simulink subsystem "flag_LiDAR_online"  (R2024a)
settings: Solver=VariableStepAuto  StartTime=0.0  StopTime=10.0  RelTol=1e-3
settings Model: Creator=gurt1  LastModifiedBy=gurt1

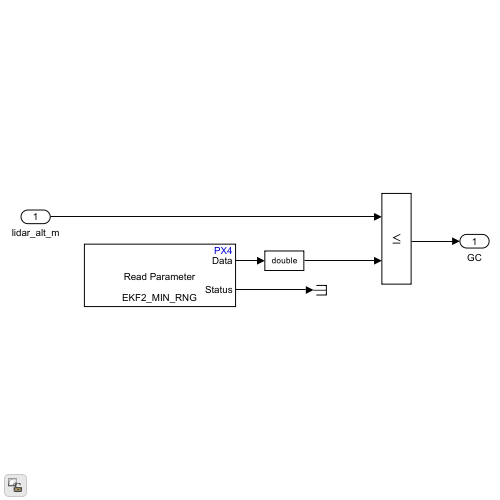
[thumbnail: Simulink's stored preview of the top-level diagram]
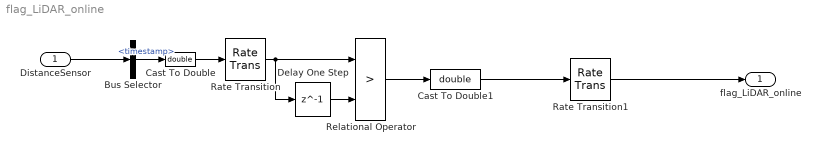
== system flag_LiDAR_online ==
  DistanceSensor : Inport
  Bus Selector : BusSelector  OutputSignals=timestamp
  Cast To Double : DataTypeConversion  OutDataTypeStr=double  SaturateOnIntegerOverflow=off  RndMeth=Floor
  Cast To Double1 : DataTypeConversion  OutDataTypeStr=double  SaturateOnIntegerOverflow=off  RndMeth=Floor
  Delay One Step : Delay  DelayLength=1
  Rate Transition : RateTransition  OutPortSampleTime=1
  Rate Transition1 : RateTransition  OutPortSampleTime=FC.samp_time
  Relational Operator : RelationalOperator  Operator=>  OutDataTypeStr=boolean  RndMeth=Simplest  InputSameDT=off
  flag_LiDAR_online : Outport
  wires:
  Cast To Double1/1 -> Rate Transition1/1
  DistanceSensor/1 -> Bus Selector/1
  Bus Selector/1 -> Cast To Double/1  "<timestamp>"
  Delay One Step/1 -> Relational Operator/2
  Cast To Double/1 -> Rate Transition/1
  Rate Transition/1 -> Delay One Step/1, Relational Operator/1
  Relational Operator/1 -> Cast To Double1/1
  Rate Transition1/1 -> flag_LiDAR_online/1
